simulink model "anav_real"  (R2018a)
settings: Solver=VariableStepAuto  StartTime=0.0  StopTime=inf  RelTol=1e-3
InitFcn:
  | run('initialize.m')
values from neighbouring files (symbols this model uses):
  limit = generateRectangle(mapDim(1)-2,mapDim(2)-2)    [initialize.m]
  mapDim = [80 40]    [buildMapTest.m]    (also in initialize.m)
  mode = 0    [initialize.m]    (also in test.m)
  sObs = nan(2, 3)    [initialize.m]
  verticies = cat(3, verticiesX, verticiesY)    [initialize.m]
undefined symbols (not defined in the file or in its folder): visualObj
settings Model: SnapshotBufferSize=5  SnapshotInterval=1  Creator=alex  LastModifiedBy=alex
settings DataIOCC: SaveOutput=off  SignalLogging=off  DSMLogging=off  SaveTime=off

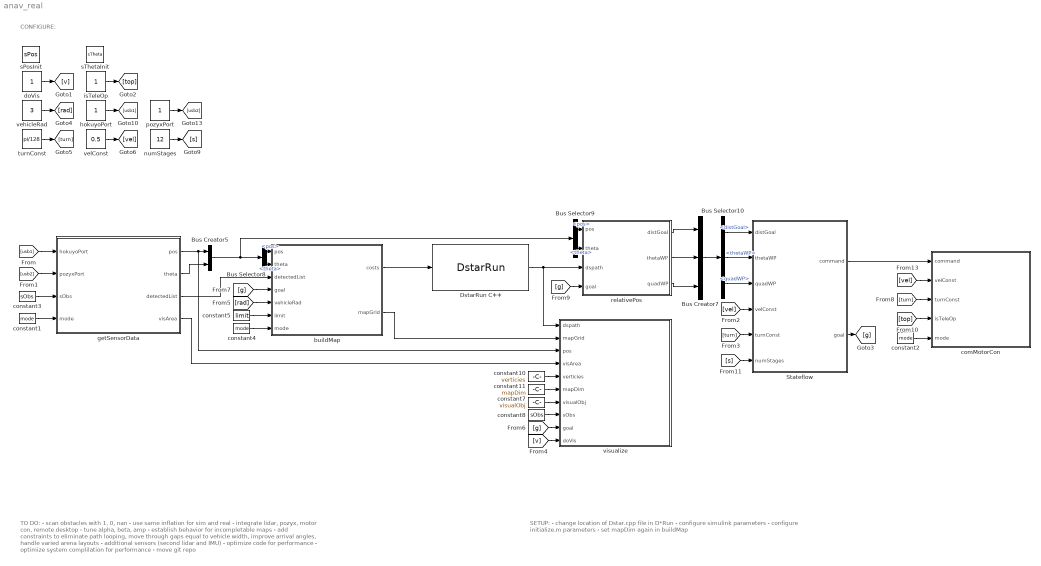
== system anav_real ==
  note: CONFIGURE:
  note: TO DO:
      | - scan obstacles with 1, 0, nan
      | - use same inflation for sim and real
      | - integrate lidar, pozyx, motor con, remote desktop
      | - tune alpha, beta, amp
      | - establish behavior for incompletable maps
      | - add constraints to eliminate path looping, move
      | through gaps equal to vehicle width, improve arrival
      | angles, handle varied arena layouts
      |
      | - additional sensors (second lidar and IMU)
      | - optimize code for performance
      | - optimize system complilation for performance
      | - move git repo
  note: SETUP:
      | - change location of Dstar.cpp file in D*Run
      | - configure simulink parameters
      | - configure initialize.m parameters
      | - set mapDim again in buildMap
  Bus Creator5 : BusCreator  Inputs=2
  Bus Creator7 : BusCreator  Inputs=3
  Bus Selector10 : BusSelector  OutputSignals=distGoal,thetaWP,quadWP
  Bus Selector8 : BusSelector  OutputSignals=pos,theta
  Bus Selector9 : BusSelector  OutputSignals=pos,theta
  DstarRun C++ : S-Function  InitFcn=try, set_param(gcb,'FunctionName','DstarRun'), end  FunctionName=DstarRun  SFunctionModules=DstarRun_wrapper Dstar  SFunctionDeploymentMode=off  EnableBusSupport=off  mask(S-Function Builder){}
      mask help: Simulink:masks:SFunctionBuilder_MD
      mask init:
      | val = [[.9  0.75 0.75 1 1 .9 .9 1]',[1 1 0.75 0.75 .9 .9 1 .9]'];try , sys = get_param(gcb,'SfunBuilderFcnName');if isempty(sys), sys = get_param(gcb,'FunctionName'); end,catch, sys = get_param(gcb,'FunctionName'); end
      settings: CopyFcn=set_param(gcbh,'LinkStatus','none')  PreSaveFcn=try, set_param(gcb,'FunctionName','DstarRun'), end  OpenFcn=sfunctionwizard(gcbh)
      mask Display: plot(val(:,1),val(:,2)),disp(sys), port_label('input',1,'costs'), port_label('output',1,'dspath')
  Stateflow : Stateflow chart  TreatAsAtomicUnit=on
  buildMap : MATLAB Function  TreatAsAtomicUnit=on
  comMotorCon : MATLAB Function  TreatAsAtomicUnit=on
  constant1 : Constant  Value=mode
  constant10 : Constant  Value=verticies  VectorParams1D=off
  constant11 : Constant  Value=mapDim  VectorParams1D=off
  constant2 : Constant  Value=mode
  constant3 : Constant  Value=sObs
  constant4 : Constant  Value=mode
  constant5 : Constant  Value=limit  VectorParams1D=off
  constant7 : Constant  Value=visualObj  VectorParams1D=off
  constant8 : Constant  Value=sObs  VectorParams1D=off
  doVis : Constant
  getSensorData : MATLAB Function  TreatAsAtomicUnit=on
  hokuyoPort : Constant
  isTeleOp : Constant
  numStages : Constant  Value=12
  pozyxPort : Constant
  relativePos : MATLAB Function  TreatAsAtomicUnit=on
  sPosInit : DataStoreMemory  DataStoreName=sPos  ReadBeforeWriteMsg=warning  WriteAfterWriteMsg=warning  WriteAfterReadMsg=warning  InitialValue=[10 10]  VectorParams1D=off  ShowAdditionalParam=off  OutDataTypeStr=double  Dimensions=[1 2]
  sThetaInit : DataStoreMemory  DataStoreName=sTheta  ReadBeforeWriteMsg=warning  WriteAfterWriteMsg=warning  WriteAfterReadMsg=warning  InitialValue=pi/4  ShowAdditionalParam=off  OutDataTypeStr=double  Dimensions=1
  turnConst : Constant  Value=pi/128
  vehicleRad : Constant  Value=3
  velConst : Constant  Value=0.5
  visualize : MATLAB Function  TreatAsAtomicUnit=on
  wires:
  isTeleOp/1 -> [top]
  vehicleRad/1 -> [rad]
  turnConst/1 -> [turn]
  velConst/1 -> [vel]
  numStages/1 -> [s]
  hokuyoPort/1 -> [usb1]
  pozyxPort/1 -> [usb2]
  [usb1] -> getSensorData/1(hokuyoPort)
  [usb2] -> getSensorData/2(pozyxPort)
  constant1/1 -> getSensorData/4(mode)
  getSensorData/1(pos) -> visualize/3(pos), Bus Creator5/1
  getSensorData/2(theta) -> Bus Creator5/2
  getSensorData/3(detectedList) -> buildMap/3(detectedList)
  [rad] -> buildMap/5(vehicleRad)
  constant4/1 -> buildMap/7(mode)
  constant5/1 -> buildMap/6(limit)
  getSensorData/4(visArea) -> visualize/4(visArea)
  buildMap/2(mapGrid) -> visualize/2(mapGrid)
  constant7/1 -> visualize/7(visualObj)
  constant8/1 -> visualize/8(sObs)
  [g] -> visualize/9(goal)
  DstarRun C++/1 -> visualize/1(dspath), relativePos/3(dspath)
  constant10/1 -> visualize/5(verticies)
  constant11/1 -> visualize/6(mapDim)
  doVis/1 -> [v]
  [v] -> visualize/10(doVis)
  buildMap/1(costs) -> DstarRun C++/1
  [g] -> relativePos/4(goal)
  Bus Selector8/1 -> buildMap/1(pos)  "<pos>"
  Bus Selector8/2 -> buildMap/2(theta)  "<theta>"
  Bus Creator5/1 -> Bus Selector9/1, Bus Selector8/1
  Bus Selector9/1 -> relativePos/1(pos)  "<pos>"
  Bus Selector9/2 -> relativePos/2(theta)  "<theta>"
  relativePos/1(distGoal) -> Bus Creator7/1
  relativePos/3(quadWP) -> Bus Creator7/3
  relativePos/2(thetaWP) -> Bus Creator7/2
  Stateflow/2(goal) -> [g]
  Stateflow/1(command) -> comMotorCon/1(command)
  constant2/1 -> comMotorCon/5(mode)
  [top] -> comMotorCon/4(isTeleOp)
  Bus Creator7/1 -> Bus Selector10/1
  constant3/1 -> getSensorData/3(sObs)
  [turn] -> comMotorCon/3(turnConst)
  [vel] -> comMotorCon/2(velConst)
  Bus Selector10/1 -> Stateflow/1(distGoal)  "<distGoal>"
  Bus Selector10/3 -> Stateflow/3(quadWP)  "<quadWP>"
  [turn] -> Stateflow/5(turnConst)
  [vel] -> Stateflow/4(velConst)
  [s] -> Stateflow/6(numStages)
  [g] -> buildMap/4(goal)
  Bus Selector10/2 -> Stateflow/2(thetaWP)  "<thetaWP>"

== matlab function anav_real/getSensorData ==
  data: hokuyoPort input; pozyxPort input; sObs input; mode input; pos output; theta output; detectedList output; visArea output; sPos data_store_memory; sTheta data_store_memory
function [pos, theta, detectedList, visArea] = getSensorData(hokuyoPort, pozyxPort, sObs, mode) 
    coder.extrinsic('tic')
    coder.extrinsic('toc')
    toc
    tic
    
    pos = [0 0];
    theta = 0;
    
    %% Real position and orientation 
    % position vector and orientation value from Pozyx
    if mode == 3
        
    end
    
    %% Simulation position and orientation 
    % starting position and orientation from simulink config
    global sPos sTheta   

    if mode == 1 || mode == 2
        % update simulation position and theta 
        pos = sPos;
        theta = sTheta;
    end
    
    %% Create vision area visual object 
    if mode == 1
        % visArea opening angle above/below horizontal and leg length 
        coneAngle = pi/4;
        coneDepth = 10;
        
        % 4 points to make visArea in polar rotated to current theta  
        t = [0 coneAngle -coneAngle 0] + theta;
        r = [0 coneDepth coneDepth 0];
        
        % convert to cartesian, z column for compatability with built-in trig 
        [x, y] = pol2cart(t, r);
        z = zeros(1,4);
        
        % list format and translate to current pos 
        visArea = rot90(vertcat(z,y,x),3);
        visArea(:,1) = visArea(:,1) + pos(1);
        visArea(:,2) = visArea(:,2) + pos(2);
    else
        % blind spot 
        visArea = zeros(4,3);
        
    end
    
    %% Real obstacle detection
    % lidar scan list from Hokuyo UTM-30LX
    nPoints = 1081;
    if mode == 2 || mode == 3
        
    end
    
    %% Simulation obstacle detection 
    detectedList = repmat([nan nan], nPoints, 1); 
        
    if mode == 1
        % get detected vector 
        sObsList = reshape(permute(sObs,[2,1,3]),size(sObs,2),[])';
        detected = detectRotated(sObsList, visArea);

        % list obstacles that are detected 
        if any(detected)
            detectedListTemp2 = repmat([nan nan], nPoints, 1); 

            sObsListX = sObsList(:,1);
            sObsListY = sObsList(:,2);
            detectedListX = sObsListX(detected==1);
            detectedListY = sObsListY(detected==1);
            detectedListTemp1 = horzcat(detectedListX, detectedListY);
            detectedListTemp2(:) = vertcat(detectedListTemp1,...
                repmat([nan nan], nPoints-size(detectedListTemp1, 1), 1));
            detectedList = detectedListTemp2;
        end
    end
end

== matlab function anav_real/relativePos ==
  data: pos input size=[1 2]; theta input; dspath input; distGoal output; goal input size=[1 2]; thetaWP output; quadWP output
function [distGoal, thetaWP, quadWP] = relativePos(pos, theta, dspath, goal)
    % theta between current orientation and line from current to waypoint 
    wayPoint = 3;
    thetaWP = radToWay(dspath(wayPoint,:), pos, theta); 
    
    % distance between pos and goal
    distGoal = distToWay(goal, pos);
    
    % quadrant of waypoint as if pos is the origin 
    quadWP = 0;
    if dspath(wayPoint, 1) >= pos(1) && dspath(wayPoint, 2) >= pos(2)
        quadWP = 1;
    elseif dspath(wayPoint, 1) < pos(1) && dspath(wayPoint, 2) >= pos(2)
        quadWP = 2;
    elseif dspath(wayPoint, 1) < pos(1) && dspath(wayPoint, 2) < pos(2)
        quadWP = 3;
    elseif dspath(wayPoint, 1) >= pos(1) && dspath(wayPoint, 2) < pos(2)
        quadWP = 4;
    end
end

== matlab function anav_real/visualize ==
  data: dspath input; mapGrid input size=[mapDim(2)-1 mapDim(1)-1]; pos input; visArea input; verticies input; mapDim input; visualObj input; sObs input; goal input; doVis input
function visualize(dspath, mapGrid, pos, visArea, verticies, mapDim, visualObj,...
                                                        sObs, goal, doVis)   
    if doVis
        %% Clear figure and set z constant above max height of surface grid 
        clf
        z = 1.1; % could be any value > 1

        %% Zeros fill extra row and column of surface grid for accurate visualization
        mapGrid = vertcat(mapGrid, zeros(1, size(mapGrid,2)));
        mapGrid = horzcat(mapGrid, zeros(size(mapGrid,1), 1));
        
        %% Set grid parameters 
        hold on; grid on; grid minor; view(0, 90)
        xlim([-1 mapDim(1)+1]); ylim([-1 mapDim(2)+1])
        xlabel('Field Length (x10 cm)'); ylabel('Field Width (x10 cm)')
        title('2D Autonomous Navigation And Obstacle Avoidance - VT 2019')
        
        %% Plotting key data and apply settings per object 
        surf(verticies(:,:,1), verticies(:,:,2), mapGrid,'EdgeColor', [0.5 0.5 0.5])
        plot3(pos(1), pos(2), z, 'o', 'MarkerSize', 15, 'MarkerEdgeColor', [0 0 0],'MarkerFaceColor', [1 1 1])
        plot3(goal(1), goal(2), z, 'p', 'MarkerSize', 20, 'MarkerEdgeColor', [1 0 0], 'MarkerFaceColor', [1 .6 .6])
        plot3(visArea(:,1), visArea(:,2), z*ones(size(visArea, 1), 1), 'y-', 'LineWidth', 3)
        plot3(dspath(:,1), dspath(:,2), z*ones(size(dspath, 1), 1), 'go-', 'LineWidth', 3, 'MarkerSize', 5)
        plot3([pos(1) dspath(3, 1)], [pos(2) dspath(3, 2)], [z z], 'k', 'LineWidth', 2);
        for i = 1:size(sObs, 3)
            plot3(sObs(:,1,i), sObs(:,2,i), z*ones(size(sObs, 1), 1), 'LineWidth', 3)
            if i <= size(visualObj, 3)
                plot3(visualObj(:,1,i), visualObj(:,2,i), z*ones(size(visualObj, 1), 1), 'r-', 'LineWidth', 3)
            end
        end         
        hold off
    end
end

== stateflow chart anav_real/Stateflow ==
  settings: stateMachineType=MOORE_MACHINE
  state change_goal
    state to_bin
      goal = bin;
      dir = b;
    state to_mine
      goal = mine;
      dir = f;
    state to_home_out
      goal = home_out;
      dir = f;
    state to_home_in
      goal = home_in;
      dir = f;
    (junction 345) -> to_bin [order 2] : [goal(2) == home_in(2)]
    (junction 345) -> to_mine [order 3] : [goal(2) == home_out(2)]
    (junction 345) -> to_home_in [order 1] : [goal(2) == mine(2)]
    (junction 345) -> to_home_out [order 4] : [goal(2) == bin(2)]
  state end
    command = 0;
  state ideal_path
    state forward_ideal
      command = 1;
    state cc_to_ideal
      command = 3;
    state cw_to_ideal
      command = 4;
    state backwards_ideal
      command = 2;
    cc_to_ideal -> (junction 243) [order 2]
    forward_ideal -> (junction 243) [order 3]
    (junction 265) -> cc_to_ideal [order 1] : [thetaWP>=0]
    (junction 243) -> (junction 265) [order 2] : [(dir == f & (quadWP == 2 | quadWP == 3))...
        | | (dir == b & (quadWP == 1 | quadWP == 4)) ]
    (junction 265) -> cw_to_ideal [order 2] : [thetaWP<0]
    (junction 261) -> cc_to_ideal [order 2] : [thetaWP<0]
    cw_to_ideal -> (junction 243) [order 2]
    (junction 243) -> (junction 261) [order 1] : [(dir == f & (quadWP == 1 | quadWP == 4))...
        | | (dir == b & (quadWP == 2 | quadWP == 3)) ]
    backwards_ideal -> (junction 243) [order 3]
    (junction 261) -> cw_to_ideal [order 1] : [thetaWP>=0]
  state goal_reached
    command = 0;
    stage = stage + 1;
  state start
    mine = [50 30];
    home_in = [7 15];
    home_out = [7 14];
    bin = [7 7];
    f = 0;
    b = pi;
    %%%%%%%%%
    dir = f;
    stage = 1;
    goal = mine;
  to_bin -> (junction 361)
  to_mine -> (junction 361)
  (junction 283) -> (junction 345) [order 2]
  to_home_out -> (junction 361)
  (junction 361) -> (junction 394)
  to_home_in -> (junction 361)
  (junction 283) -> end [order 1] : [stage > numStages]
  (junction 375) -> (junction 211) [order 1] : [(dir == f & (quadWP == 2 | quadWP == 3))...
      | | (dir == b & (quadWP == 1 | quadWP == 4)) ]
  (junction 211) -> (junction 161) : [(thetaWP < pi & thetaWP  > pi-turnConst)...
      | | (thetaWP  >= -pi & thetaWP  < -pi+turnConst)]
  goal_reached -> (junction 283)
  (junction 161) -> (junction 399) [order 2]
  (junction 375) -> (junction 209) [order 2] : [(dir == f & (quadWP == 1 | quadWP == 4))...
      | | (dir == b & (quadWP == 2 | quadWP == 3)) ]
  (junction 209) -> (junction 161) : [(thetaWP  >= -turnConst & thetaWP  < turnConst)]
  (junction 183) -> (junction 375)
  (junction 161) -> (junction 382) [order 1]
  forward_ideal -> (junction 183) [order 2]
  (junction 377) -> goal_reached : [distGoal < velConst]
  forward_ideal -> (junction 377) [order 1]
  (junction 382) -> forward_ideal [order 1] : [dir == f]
  cc_to_ideal -> (junction 183) [order 1]
  (junction 394) -> (junction 243)
  cw_to_ideal -> (junction 183) [order 1]
  (junction 382) -> backwards_ideal [order 2] : [dir == b]
  backwards_ideal -> (junction 183) [order 2]
  backwards_ideal -> (junction 377) [order 1]
  (default) -> start
  start -> (junction 394)
  data: distGoal input; thetaWP input; quadWP input; velConst input; command output; goal output; mine local double size=[1 2]; home_in local double size=[1 2]; bin local double size=[1 2]; home_out local double size=[1 2]; dir local double size=1; f local double size=1; b local double size=1; stage local double size=1; turnConst input; numStages input

== matlab function anav_real/comMotorCon ==
  data: command input; velConst input; turnConst input; isTeleOp input; mode input; sPos data_store_memory; sTheta data_store_memory
function comMotorCon(command, velConst, turnConst, isTeleOp, mode)   
    %% Send commands to motor controller 
    if mode == 2 || mode == 3
        
    end
    
    %% Get start/stop and takeover commands from tele op 
    if isTeleOp == 1 && (mode == 2 || mode == 3)
        
    end
    
    %% Update simulation position and theta 
    global sPos sTheta
    
    if mode == 1
        if command == 0
            % do nothing 
        elseif command == 1
            % forward
            sPos(1) = sPos(1) + velConst*cos(sTheta);
            sPos(2) = sPos(2) + velConst*sin(sTheta);
        elseif command == 2
            % backwards
            sPos(1) = sPos(1) - velConst*cos(sTheta);
            sPos(2) = sPos(2) - velConst*sin(sTheta);
        elseif command == 3
            % counter clockwise
            sTheta = sTheta + turnConst;
        elseif command == 4
            % clockwise 
            sTheta = sTheta - turnConst;
        end  
    end
end

== matlab function anav_real/buildMap ==
  data: pos input; costs output; theta input; detectedList input; goal input; vehicleRad input; limit input; mode input; mapGrid output size=[mapDim(2)-1 mapDim(1)-1]
function [costs, mapGrid] = buildMap(pos, theta, detectedList, goal, vehicleRad,...
                                        limit, mode)
    mapDim = [58 37]; % must be equalivant in initialize.m
    
    persistent mapGridP
    
    if isempty(mapGridP)
        mapGridP = zeros(mapDim(2)-1, mapDim(1)-1);
    end
    
    %% Orient polar list 
    if mode == 2 || mode == 3
        
    end
    
    %% Translate cartesian list 
    if mode == 2 || mode == 3
        
    end
    
    %% Add limit and inflate points
    if mode == 1
        % inflate dcm n = ~500 and use rounding 
        detectedLimitList = vertcat(limit(:,1:2), detectedList);
        inflated = inflate(detectedLimitList, vehicleRad, mode);
    else
        % inflate mm n = ~100 and dont use rounding (find alternative)
        inflated = 0;
        
    end
    
    %% Eliminate points outside limit 
    if mode == 1
        inflated(inflated(:, 1) <= 0, :) = [];
        inflated(inflated(:, 1) >= mapDim(1), :) = [];
        inflated(inflated(:, 2) <= 0, :) = [];
        inflated(inflated(:, 2) >= mapDim(2), :) = [];
    else
        % scale size for real
        inflated(inflated(:, 1) <= 0, :) = [];
        inflated(inflated(:, 1) >= mapDim(1), :) = [];
        inflated(inflated(:, 2) <= 0, :) = [];
        inflated(inflated(:, 2) >= mapDim(2), :) = [];
    end

    %% Convert list to grid 
    if mode == 1
        mapGridNew = list2grid(inflated(:,1), inflated(:,2), mapDim(1)-1, mapDim(2)-1);
    else 
        % scale size for real
        mapGridNew = list2grid(inflated(:,1), inflated(:,2), mapDim(1)-1, mapDim(2)-1);
    end
    
    %% Compress 1e-3 m grid to 1e-1 m grid
    if mode == 2 || mode == 3
        
    end
    
    %% Persist grid and average with new 
    alpha = 0.99; beta = 0.01;
    mapGridP = alpha*mapGridP + beta*mapGridNew;
    mapGrid = mapGridP;
    
    %% Convert probability grid to list for d*
    mapList = grid2list(mapGrid);
    % convert into 1-by vector: size pos goal mapList1:end
    costsTemp = vertcat([numel(mapList)/3 0 0], [pos 0], [goal 0], mapList);
    costs = reshape(costsTemp.',1,numel(costsTemp));
end
